simulink model "chirp_excite_controlled"  (R2012b)
settings: Solver=FixedStepDiscrete  StartTime=0.0  StopTime=Tfinal  RelTol=1e-3
undefined symbols (not defined in the file or in its folder): GAIN, Kd, KON, National_Instruments, PCI, Tfinal, Ts
libraries: rtwinlib x2, simulink x1, dspsrcs4 x1
settings Model: SimulationMode=external  ExtModeTrigDuration=1000000  ExtModeArchiveMode=auto  ExtModeArchiveFileName=dataarch  ExtModeArchiveDirName=.\  Creator=f.cardoso-ribeiro  LastModifiedBy=f.cardoso-ribeiro
settings SolverCC: AutoInsertRateTranBlk=on
settings DataIOCC: LimitDataPoints=off  SaveOutput=off  SignalLogging=off  DSMLogging=off  SaveTime=off
settings HardwareCC: ProdIntDivRoundTo=Zero  ProdEndianess=LittleEndian  ProdHWDeviceType=Generic->32-bit x86 compatible
settings RTWCC: SystemTargetFile=rtwin.tlc  TemplateMakefile=rtwin.tmf  Description=Real-Time Windows Target  RTWVerbose=off  ProcessScript=rtwin_make_rtw_hook  RTWCompilerOptimization=On
settings CodeAppCC: MaxIdLength=95
settings RTWinTargetCC: TargetLibSuffix=_rtwin.lib  TargetPreCompLibLocation=C:\Program Files\MATLAB\R2012b\toolbox\rtw\targets\rtwin\lib\win64  CodeReplacementLibrary=ANSI_C  RTWinDir=C:/PROGRA~1/MATLAB/R2012b/toolbox/rtw/targets/rtwin  TargetArch=win64

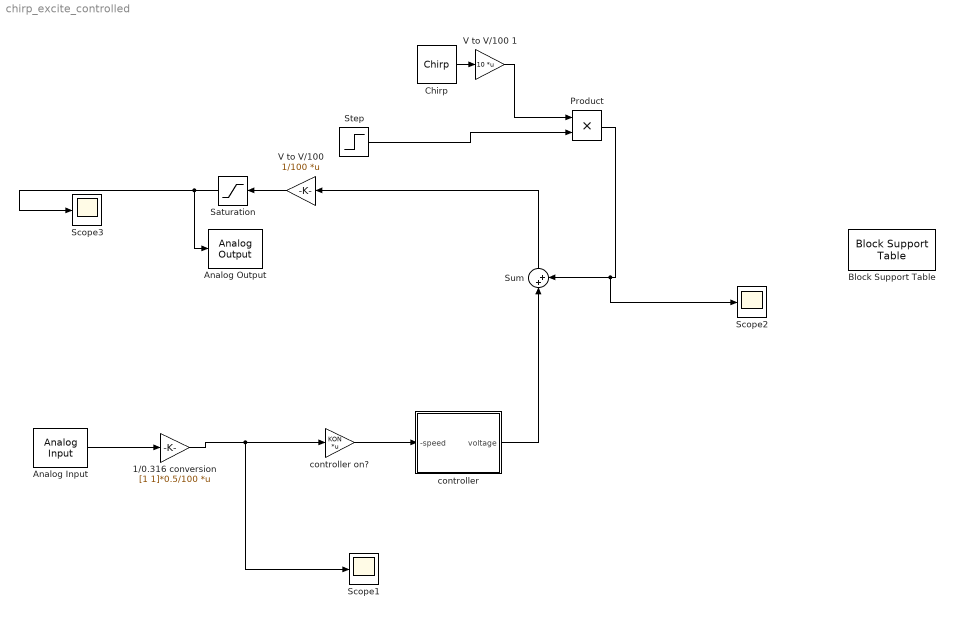
== system chirp_excite_controlled ==
  1/0.316 conversion : Gain  Gain=[1 1]*0.5/100  Multiplication=Matrix(K*u)
  Analog Input : rtwinlib/Analog Input  SampleTime=Ts  MaxMissedTicks=10  ShowMissedTicks=off  YieldWhenWaiting=off  DrvName=National_Instruments/PCI-6024E  DrvAddress=4294967295  DrvOptions=[1 0 0 0 0 0]  Channels=[1 2]  RangeMode=1  VoltRange=2  DataType=1
      settings: AttributesFormatString=National Instruments\nPCI-6024E [auto]
  Analog Output : rtwinlib/Analog Output  SampleTime=Ts  MaxMissedTicks=10  ShowMissedTicks=off  YieldWhenWaiting=off  DrvName=National_Instruments/PCI-6024E  DrvAddress=4294967295  DrvOptions=[1 0 0 0 0 0]  Channels=[1 2]  RangeMode=1  VoltRange=1  InitialValue=0  FinalValue=0
      settings: AttributesFormatString=National Instruments\nPCI-6024E [auto]
  Block Support Table : simulink/Model-Wide Utilities/Block Support Table
  Chirp : dspsrcs4/Chirp  sweep=Logarithmic  mode=Unidirectional  f0=1  f1=40  t1=tf  Tsweep=tf  phase=0  Ts=Ts  spf=1  datatype=Double
  Product : Product  RndMeth=Zero
  Saturation : Saturate  UpperLimit=1.5  LowerLimit=-1.5
  Scope1 : Scope
      settings: TimeRange=60  YMin=-0.025  YMax=0.025  SaveName=output
  Scope2 : Scope
      settings: YMin=-10  YMax=10  SaveName=input
  Scope3 : Scope
      settings: TimeRange=240  YMin=-0.12  YMax=0.12  SaveName=control_input
  Step : Step  Time=Tfinal-20  Before=1  After=0  SampleTime=0
  Sum : Sum  Inputs=|++
  "V to V/100 " : Gain  Gain=1/100  Multiplication=Matrix(K*u)
  V to V/100 1 : Gain  Gain=10  Multiplication=Matrix(K*u)
  controller : Subsystem
  controller on? : Gain  Gain=KON  Multiplication=Matrix(K*u)
  wires:
  Analog Input/1 -> 1/0.316 conversion/1
  "V to V/100 "/1 -> Saturation/1
  controller on?/1 -> controller/1(-speed)
  controller/1(voltage) -> Sum/1
  Step/1 -> Product/2
  Sum/1 -> "V to V/100 "/1
  Product/1 -> Scope2/1, Sum/2
  Saturation/1 -> Analog Output/1, Scope3/1
  1/0.316 conversion/1 -> Scope1/1, controller on?/1
  Chirp/1 -> V to V/100 1/1
  V to V/100 1/1 -> Product/1

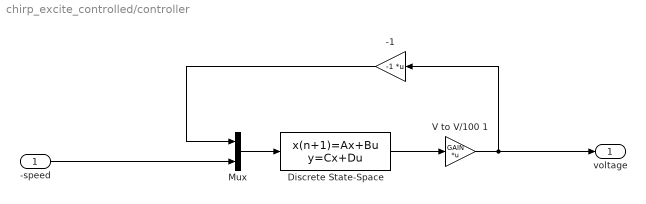
== system chirp_excite_controlled/controller ==
  -speed : Inport
  -1 : Gain  Gain=-1  Multiplication=Matrix(K*u)
  Discrete State-Space : DiscreteStateSpace  A=Kd.a  B=Kd.b  C=Kd.c  D=Kd.d  SampleTime=-1
  Mux : Mux  Inputs=2
  V to V/100 1 : Gain  Gain=GAIN  Multiplication=Matrix(K*u)
  voltage : Outport
  wires:
  -1/1 -> Mux/1
  V to V/100 1/1 -> voltage/1, -1/1
  Discrete State-Space/1 -> V to V/100 1/1
  -speed/1 -> Mux/2
  Mux/1 -> Discrete State-Space/1
